simulink model "Collision_avoidance"  (R2020a)
settings: Solver=FixedStepAuto  StartTime=0.0  StopTime=inf  RelTol=1e-3
model workspace (MAT data in the model file):
  SL_ROS_VariableLengthArrays_MaxSizes.CommonInfo.ArrayTruncateAction = 'EmitWarning'
  SL_ROS_VariableLengthArrays_MaxSizes.MsgTypeMap = containers.Map
  SL_ROS_VariableLengthArrays_MaxSizes.MsgTypeMap.serialization.keys = {'sensor_msgs/CompressedImage', 'sensor_msgs/LaserScan'}
  SL_ROS_VariableLengthArrays_MaxSizes.MsgTypeMap.serialization.values{1}(1).PropertyName = 'Data'
  SL_ROS_VariableLengthArrays_MaxSizes.MsgTypeMap.serialization.values{1}(1).DataType = 'uint8'
  SL_ROS_VariableLengthArrays_MaxSizes.MsgTypeMap.serialization.values{1}(1).MaxLength = 200000
  SL_ROS_VariableLengthArrays_MaxSizes.MsgTypeMap.serialization.values{1}(2).PropertyName = 'Format'
  SL_ROS_VariableLengthArrays_MaxSizes.MsgTypeMap.serialization.values{1}(2).DataType = 'uint8'
  SL_ROS_VariableLengthArrays_MaxSizes.MsgTypeMap.serialization.values{1}(2).MaxLength = 128
  SL_ROS_VariableLengthArrays_MaxSizes.MsgTypeMap.serialization.values{2}(1).PropertyName = 'Intensities'
  SL_ROS_VariableLengthArrays_MaxSizes.MsgTypeMap.serialization.values{2}(1).DataType = 'single'
  SL_ROS_VariableLengthArrays_MaxSizes.MsgTypeMap.serialization.values{2}(1).MaxLength = 360
  SL_ROS_VariableLengthArrays_MaxSizes.MsgTypeMap.serialization.values{2}(2).PropertyName = 'Ranges'
  SL_ROS_VariableLengthArrays_MaxSizes.MsgTypeMap.serialization.values{2}(2).DataType = 'single'
  SL_ROS_VariableLengthArrays_MaxSizes.MsgTypeMap.serialization.values{2}(2).MaxLength = 360
  SL_ROS_VariableLengthArrays_MaxSizes.MsgTypeMap.serialization.uniformity = 0
  SL_ROS_VariableLengthArrays_MaxSizes.MsgTypeMap.serialization.keyType = 'char'
  SL_ROS_VariableLengthArrays_MaxSizes.MsgTypeMap.serialization.valueType = 'any'
undefined symbols (not defined in the file): Angular, freq, Linear, steering_rate_limit
libraries: simulink_extras x5, robotlib x4, simulink x2, realtime_pacer_lib x2, sharedtransform x1, visiongeotforms x1, drivingvehiclecontroller x1, visionsinks x1
settings Model: Creator=20195009  LastModifiedBy=TruckLabPC2
settings OptimizationCC: EnhancedBackFolding=on  PassReuseOutputArgsAs=Individual arguments  ZeroExternalMemoryAtStartup=off  ZeroInternalMemoryAtStartup=off  MaxStackSize=64  OptimizeBlockOrder=speed  DifferentSizesBufferReuse=on  OptimizationCustomize=off  EfficientTunableParamExpr=on
settings DebuggingCC: ParameterTunabilityLossMsg=error  SFMachineParentedDataDiag=error
settings HardwareCC: ProdBitPerPointer=32  ProdBitPerSizeT=32  ProdBitPerPtrDiffT=32  ProdLargestAtomicFloat=None  ProdIntDivRoundTo=Undefined  ProdEndianess=Unspecified  ProdWordSize=32  ProdHWDeviceType=Generic->Unspecified (assume 32-bit Generic)
settings SFSimCC: MATLABDynamicMemAlloc=off
settings RTWCC: SystemTargetFile=ert.tlc  HardwareBoard=Robot Operating System (ROS)  TemplateMakefile=ert_default_tmf  Toolchain=Catkin  TargetLang=C++
settings CodeAppCC: ForceParamTrailComments=on  IgnoreCustomStorageClasses=off  OperatorAnnotations=on  SimulinkDataObjDesc=on  SFDataObjDesc=on  InsertBlockDesc=on

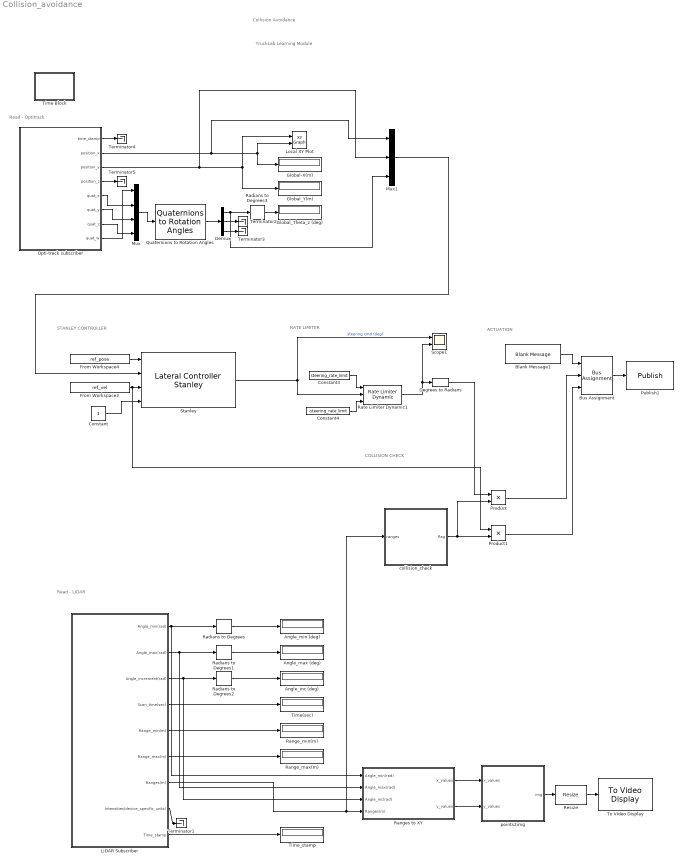
== system Collision_avoidance ==
  note: COLLISION CHECK
  note: ACTUATION
  note: RATE LIMITER
  note: STANLEY CONTROLLER
  note: Read - Optitrack
  note: TruckLab Learning Module
  note: Collision Avoidance
  note: Read - LiDAR
  Angle_inc (deg) : Display
  Angle_max (deg) : Display
  Angle_min (deg) : Display
  Blank Message1 : robotlib/Blank Message  messageClass=Message  entityType=geometry_msgs/Twist  messageType=geometry_msgs/Twist  SampleTime=1/freq
  Bus Assignment : BusAssignment  DialogController=Simulink.DDGSource_BusAssignment  AssignedSignals=Angular.Z,Linear.X
  Constant : Constant
  Constant3 : Constant  Value=steering_rate_limit
  Constant4 : Constant  Value=-steering_rate_limit
  Degrees to Radians : simulink_extras/Transformations/Degrees to Radians
  Demux : Demux  Outputs=3
  From Workspace2 : FromWorkspace  VariableName=ref_vel
  From Workspace4 : FromWorkspace  VariableName=ref_pose
  Global-X(m) : Display
  Global_Theta_z (deg) : Display
  Global_Y(m) : Display
  LiDAR Subscriber : Subsystem
  Local XY Plot : simulink/Sinks/XY Graph  xmin=0  xmax=6  ymin=0  ymax=6  st=-1
  Mux : Mux
  Mux1 : Mux  Inputs=3
  Opti-track subscriber : Subsystem
  Product : Product
  Product1 : Product
  Publish1 : robotlib/Publish  topicSource=Specify your own  topic=/tractor1/cmd_tractor1  messageType=geometry_msgs/Twist  messageQueueLength=1
      link override SinkBlock: ROSTopic=/cmd_vel  ROSMessageType=geometry_msgs/Twist  SLBusName=SL_Bus_TruckLab_MannualDrivingROS1_geometry_msgs_Twist  ModelName=TruckLab_MannualDrivingROS1  BlockId=Pub_TruckLab_MannualDrivingROS1_402
  Quaternions to Rotation Angles : sharedtransform/Quaternions to Rotation Angles  rotationOrder=ZXY  aMode=aMode
      settings: SourceProductBaseCode=AE,PW,MT,VE,VP
  Radians to Degrees{,1..3} (4 alike) : simulink_extras/Transformations/Radians to Degrees
  Range_max(m) : Display
  Range_min(m) : Display
  Ranges to XY : Subsystem
  Rate Limiter Dynamic1 : simulink/Discontinuities/Rate Limiter Dynamic
  Resize : visiongeotforms/Resize  specify=Output size as a percentage of input size  rfactor=[100 100]  outCols=25  outRows=25  outRowsCols=[25 35]  interp_method=Bilinear  antialias=on  useROI=off  roiFlag=off  roundingMode=Nearest  overflowMode=on  prodOutputMode=Binary point scaling  prodOutputWordLength=32  prodOutputFracLength=10
      settings: SourceProductBaseCode=VP
  Scope1 : Scope  NumInputPorts=2
  Stanley : drivingvehiclecontroller/Lateral Controller Stanley  ModelType=Kinematic bicycle model  PositionGainF=ref_Kf  PositionGainR=ref_Kr  YawRateGain=0.2  DelayGain=0.2  VehicleMass=1575  Lf=1.2  Lr=1.6  TireStiffness=19000  Wheelbase=0.272  MaxSteeringAngle=25
      settings: SourceProductBaseCode=DR
  Terminator{1..5} (5 alike) : Terminator
  Time Block : Subsystem
  Time(sec) : Display
  Time_stamp : Display
  To Video Display : visionsinks/To Video Display  windowSizeMode=True size (1:1)  openAtMdlStart=on  fullScreen=off  videoWindowX=817  videoWindowY=234  saveWindowSize=off  videoWindowWidth=800  videoWindowHeight=800  inputColorFormat=RGB  inputType=Obsolete  imagePorts=One multidimensional signal  OutputDevice=On-screen video monitor  dataOrg=Column-major  isWindowOpen=off
  collision_check : MATLAB Function  TreatAsAtomicUnit=on
  points2img : MATLAB Function  TreatAsAtomicUnit=on
  wires:
  Opti-track subscriber/3(position_y) -> Global_Y(m)/1, Local XY Plot/1, Mux1/2
  Opti-track subscriber/2(position_x) -> Mux1/1, Global-X(m)/1, Local XY Plot/2
  Mux/1 -> Quaternions to Rotation Angles/1
  Quaternions to Rotation Angles/1 -> Demux/1
  Demux/1 -> Mux1/3, Radians to Degrees3/1
  Radians to Degrees3/1 -> Global_Theta_z (deg)/1
  Demux/2 -> Terminator2/1
  Demux/3 -> Terminator3/1
  Opti-track subscriber/5(quat_x) -> Mux/2
  Opti-track subscriber/6(quat_y) -> Mux/3
  Opti-track subscriber/7(quat_z) -> Mux/4
  Opti-track subscriber/8(quat_w) -> Mux/1
  Opti-track subscriber/1(time_stamp) -> Terminator4/1
  Opti-track subscriber/4(position_z) -> Terminator5/1
  Constant/1 -> Stanley/4
  From Workspace4/1 -> Stanley/1
  Mux1/1 -> Stanley/2
  Stanley/1 -> Rate Limiter Dynamic1/2, Scope1/1  "steering cmd (deg)"
  From Workspace2/1 -> Product1/1, Stanley/3
  Blank Message1/1 -> Bus Assignment/1
  Bus Assignment/1 -> Publish1/1
  Degrees to Radians/1 -> Product/1
  Constant4/1 -> Rate Limiter Dynamic1/3
  Constant3/1 -> Rate Limiter Dynamic1/1
  Rate Limiter Dynamic1/1 -> Scope1/2, Degrees to Radians/1
  LiDAR Subscriber/7(Ranges(m)) -> collision_check/1(ranges), Ranges to XY/4(Ranges(m))
  LiDAR Subscriber/4(Scan_time(sec)) -> Time(sec)/1
  Radians to Degrees1/1 -> Angle_max (deg)/1
  LiDAR Subscriber/3(Angle_increment(rad)) -> Radians to Degrees2/1, Ranges to XY/3(Angle_inc(rad))
  Radians to Degrees/1 -> Angle_min (deg)/1
  Ranges to XY/1(x_values) -> points2img/1(x_values)
  LiDAR Subscriber/8(Intensities(device_specific_units)) -> Terminator1/1
  LiDAR Subscriber/2(Angle_max(rad)) -> Radians to Degrees1/1, Ranges to XY/2(Angle_max(rad))
  LiDAR Subscriber/1(Angle_min(rad)) -> Ranges to XY/1(Angle_min(rad)), Radians to Degrees/1
  LiDAR Subscriber/6(Range_max(m)) -> Range_max(m)/1
  LiDAR Subscriber/9(Time_stamp) -> Time_stamp/1
  points2img/1(img) -> Resize/1
  Radians to Degrees2/1 -> Angle_inc (deg)/1
  Resize/1 -> To Video Display/1
  LiDAR Subscriber/5(Range_min(m)) -> Range_min(m)/1
  Ranges to XY/2(y_values) -> points2img/2(y_values)
  collision_check/1(flag) -> Product/2, Product1/2
  Product/1 -> Bus Assignment/2
  Product1/1 -> Bus Assignment/3

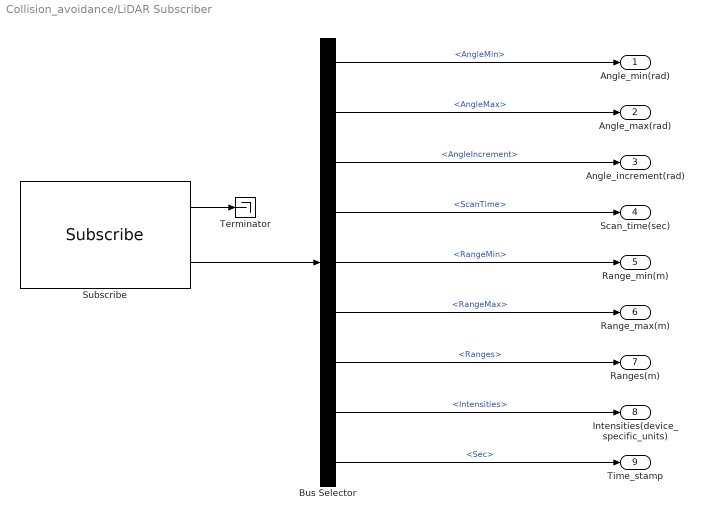
== system Collision_avoidance/LiDAR Subscriber ==
  Bus Selector : BusSelector  OutputSignals=AngleMin,AngleMax,AngleIncrement,ScanTime,RangeMin,RangeMax,Ranges,Intensities,Header.Stamp.Sec
  Subscribe : robotlib/Subscribe  topicSource=Select from ROS network  topic=/DC_1/TRACTOR_1/LIDAR_1/lidarscanfull  messageType=sensor_msgs/LaserScan  sampleTime=-1  messageQueueLength=1
  Terminator : Terminator
  Angle_min(rad) : Outport
  Angle_max(rad) : Outport  Port=2
  Angle_increment(rad) : Outport  Port=3
  Scan_time(sec) : Outport  Port=4
  Range_min(m) : Outport  Port=5
  Range_max(m) : Outport  Port=6
  Ranges(m) : Outport  Port=7
  Intensities(device_specific_units) : Outport  Port=8
  Time_stamp : Outport  Port=9
  wires:
  Subscribe/1 -> Terminator/1
  Subscribe/2 -> Bus Selector/1
  Bus Selector/1 -> Angle_min(rad)/1  "<AngleMin>"
  Bus Selector/2 -> Angle_max(rad)/1  "<AngleMax>"
  Bus Selector/5 -> Range_min(m)/1  "<RangeMin>"
  Bus Selector/6 -> Range_max(m)/1  "<RangeMax>"
  Bus Selector/8 -> Intensities(device_specific_units)/1  "<Intensities>"
  Bus Selector/9 -> Time_stamp/1  "<Sec>"
  Bus Selector/3 -> Angle_increment(rad)/1  "<AngleIncrement>"
  Bus Selector/7 -> Ranges(m)/1  "<Ranges>"
  Bus Selector/4 -> Scan_time(sec)/1  "<ScanTime>"

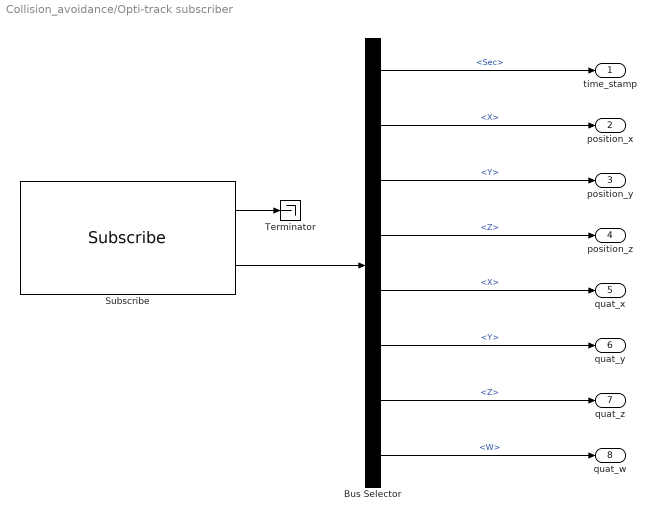
== system Collision_avoidance/Opti-track subscriber ==
  Bus Selector : BusSelector  OutputSignals=Header.Stamp.Sec,Pose.Position.X,Pose.Position.Y,Pose.Position.Z,Pose.Orientation.X,Pose.Orientation.Y,Pose.Orientation.Z,Pose.Orientation.W
  Subscribe : robotlib/Subscribe  topicSource=Select from ROS network  topic=/DC_1/TRACTOR_1/optitrack  messageType=geometry_msgs/PoseStamped  sampleTime=-1  messageQueueLength=1
  Terminator : Terminator
  time_stamp : Outport
  position_x : Outport  Port=2
  position_y : Outport  Port=3
  position_z : Outport  Port=4
  quat_x : Outport  Port=5
  quat_y : Outport  Port=6
  quat_z : Outport  Port=7
  quat_w : Outport  Port=8
  wires:
  Subscribe/1 -> Terminator/1
  Subscribe/2 -> Bus Selector/1
  Bus Selector/1 -> time_stamp/1  "<Sec>"
  Bus Selector/2 -> position_x/1  "<X>"
  Bus Selector/3 -> position_y/1  "<Y>"
  Bus Selector/4 -> position_z/1  "<Z>"
  Bus Selector/5 -> quat_x/1  "<X>"
  Bus Selector/6 -> quat_y/1  "<Y>"
  Bus Selector/7 -> quat_z/1  "<Z>"
  Bus Selector/8 -> quat_w/1  "<W>"

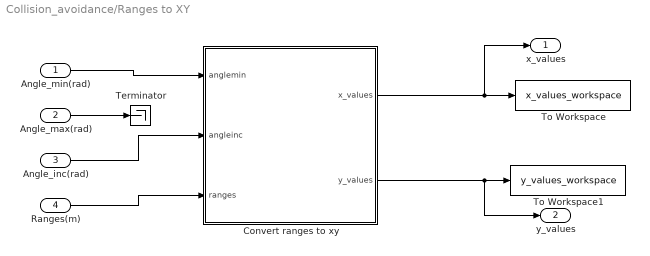
== system Collision_avoidance/Ranges to XY ==
  Angle_min(rad) : Inport
  Angle_max(rad) : Inport  Port=2
  Angle_inc(rad) : Inport  Port=3
  Ranges(m) : Inport  Port=4
  Convert ranges to xy : MATLAB Function  TreatAsAtomicUnit=on
  Terminator : Terminator
  To Workspace : ToWorkspace  VariableName=x_values_workspace  SampleTime=-1
  To Workspace1 : ToWorkspace  VariableName=y_values_workspace  SampleTime=-1
  x_values : Outport
  y_values : Outport  Port=2
  wires:
  Angle_min(rad)/1 -> Convert ranges to xy/1(anglemin)
  Angle_max(rad)/1 -> Terminator/1
  Angle_inc(rad)/1 -> Convert ranges to xy/2(angleinc)
  Ranges(m)/1 -> Convert ranges to xy/3(ranges)
  Convert ranges to xy/1(x_values) -> x_values/1, To Workspace/1
  Convert ranges to xy/2(y_values) -> y_values/1, To Workspace1/1

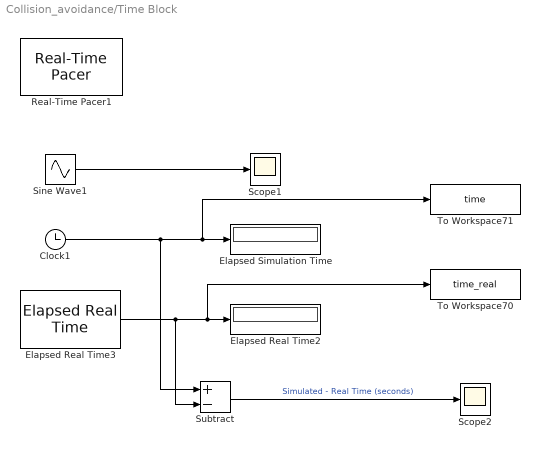
== system Collision_avoidance/Time Block ==
  Clock1 : Clock
  Elapsed Real Time2 : Display
      settings: Decimation=2
  Elapsed Real Time3 : realtime_pacer_lib/Elapsed Real Time
  Elapsed Simulation Time : Display
      settings: Decimation=2
  Real-Time Pacer1 : realtime_pacer_lib/Real-Time Pacer  simTimePerRealTime=1
  Scope1 : Scope
  Scope2 : Scope
  Sine Wave1 : Sin  Frequency=2*pi*0.5  SampleTime=0
  Subtract : Sum  Inputs=+-
  To Workspace70 : ToWorkspace  VariableName=time_real  SampleTime=-1
  To Workspace71 : ToWorkspace  VariableName=time  SampleTime=-1
  wires:
  Subtract/1 -> Scope2/1  "Simulated - Real Time (seconds)"
  Elapsed Real Time3/1 -> Elapsed Real Time2/1, To Workspace70/1, Subtract/2
  Sine Wave1/1 -> Scope1/1
  Clock1/1 -> Subtract/1, Elapsed Simulation Time/1, To Workspace71/1

== matlab function Collision_avoidance/collision_check ==
  data: flag output; ranges input
function flag = collision_check(ranges)
range_cabin = 0.2;
dist_check = 0.4;
ranges_of_interest = ranges((ranges > range_cabin) & (ranges < dist_check));
size_var = size(ranges_of_interest, 1) * size(ranges_of_interest, 2);
if size_var > 0
    flag = 0;
else
    flag = 1;
end

== matlab function Collision_avoidance/Ranges to XY/Convert ranges to xy ==
  data: anglemin input; x_values output; angleinc input; ranges input; y_values output
function [x_values, y_values] = fcn(anglemin, angleinc, ranges)
angle_min = double(anglemin);
angle_inc = double(angleinc);
angles=double(zeros(numel(ranges),1));
for i=1:numel(ranges)
    angles(i) = double(angle_min) + double(i-1)*(angle_inc);
end

x_values = ranges.*cos(angles);
y_values = ranges.*sin(angles);

== matlab function Collision_avoidance/points2img ==
  data: img output; x_values input; y_values input
function img = points2img(x_values, y_values)
img = ones(800, 800)*255;
delta = 2;
delta_ego = 5;
% iterate over these points, and set up a primitive grid map
for i=1:numel(x_values)
    % (800, 800) pixels = (8m, 8m)
    m_to_px = 100;
    x = x_values(i);
    y = y_values(i);
    
    px_x = floor(x * m_to_px);
    px_y = floor(y * m_to_px);
    
    ind_min_x = max(1, px_x-delta+400);
    ind_max_x = min(800, px_x+delta+400);
    
    ind_min_y = max(1, px_y-delta+400);
    ind_max_y = min(800, px_y+delta+400);
    
    img(ind_min_x:ind_max_x, ind_min_y:ind_max_y) = 0;
    img(400-delta_ego:400+delta_ego, 400-delta_ego:400+delta_ego) = 0;
end
